simulink model "Athena_HIL_Test_2"  (R2024b)
settings: Solver=FixedStepAuto  StartTime=0.0  StopTime=inf  FixedStep=0.001  RelTol=1e-3
undefined symbols (not defined in the file or in its folder): Payload
libraries: uavmavlinklib x4, dspnetwork x2, shared6dof x1
settings Model: Creator=ercu  LastModifiedBy=ercu

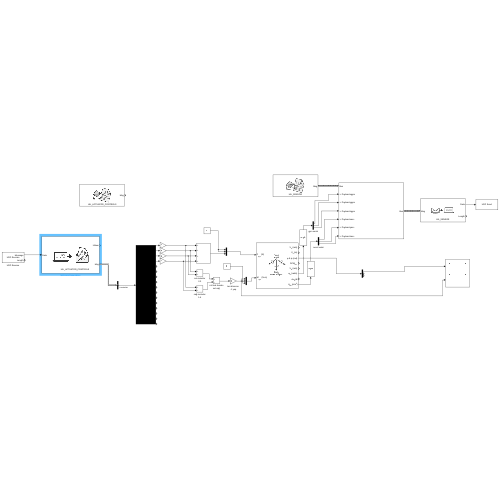
[thumbnail: Simulink's stored preview of the top-level diagram]
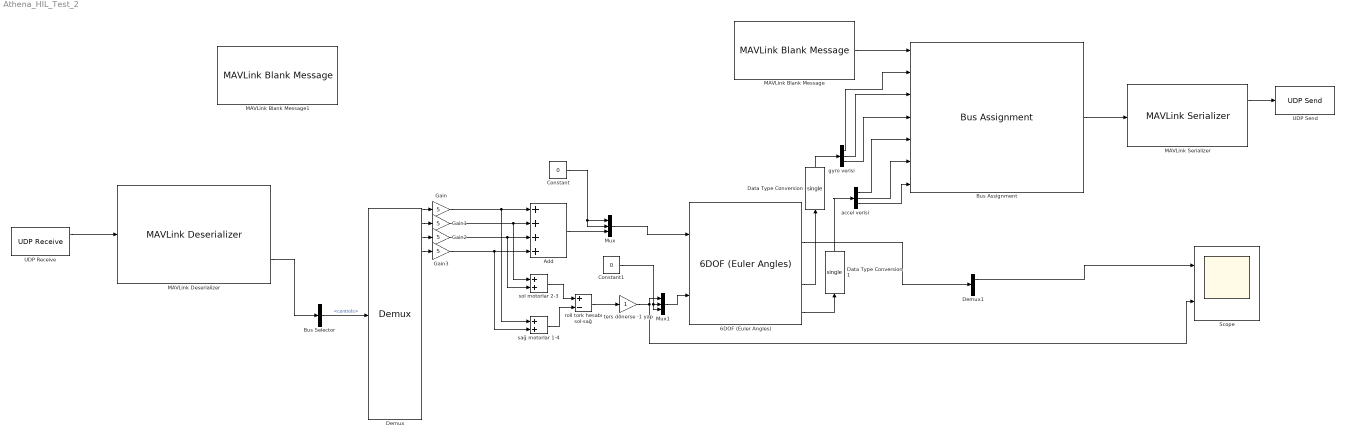
== system Athena_HIL_Test_2 ==
  6DOF (Euler Angles) : shared6dof/6DOF (Euler Angles)  units=Metric (MKS)  mtype=Fixed  rep=Euler Angles  xme_0=[0 0 -10]  Vm_0=[0 0 0]  eul_0=[0.5 0 0]  pm_0=[0 0 0]  mass_0=1.0  mass_e=0.5  mass_f=2.0  inertia=eye(3) * 0.08  inertia_e=eye(3)  inertia_f=2*eye(3)  k_quat=1.0  vre_flag=on  abi_flag=off  aMode=0  xme_statename=''  Vm_statename=''  eul_statename=''  quat_statename=''  pm_statename=''  mass_statename=''
  Add : Sum  Inputs=++++  OutDataTypeStr=double
  Bus Assignment : BusAssignment  AssignedSignals=Payload.xgyro,Payload.ygyro,Payload.zgyro,Payload.xacc,Payload.yacc,Payload.zacc
  Bus Selector : BusSelector  OutputSignals=Payload.controls
  Constant : Constant  Value=0
  Constant1 : Constant  Value=0
  Data Type Conversion : DataTypeConversion  OutDataTypeStr=single  SaturateOnIntegerOverflow=off  RndMeth=Floor
  Data Type Conversion1 : DataTypeConversion  OutDataTypeStr=single  SaturateOnIntegerOverflow=off  RndMeth=Floor
  Demux : Demux  Outputs=16
  Demux1 : Demux  Outputs=3
  Gain{,1..3} (4 alike) : Gain  Gain=5
  MAVLink Blank Message : uavmavlinklib/MAVLink Blank Message  dialectSource=Select from standard MAVLink dialects  dialect=common.xml  dialectCustom=common.xml  version=2  messageType=HIL_SENSOR  SystemID=1  ComponentID=1  SampleTime=inf
  MAVLink Blank Message1 : uavmavlinklib/MAVLink Blank Message  dialectSource=Select from standard MAVLink dialects  dialect=common.xml  dialectCustom=common.xml  version=2  messageType=HIL_ACTUATOR_CONTROLS  SystemID=1  ComponentID=1  SampleTime=inf
  MAVLink Deserializer : uavmavlinklib/MAVLink Deserializer  dialectSource=Select from standard MAVLink dialects  dialect=common.xml  dialectCustom=common.xml  version=2  messageType=HIL_ACTUATOR_CONTROLS  inputDataLength=off  SystemIDFilter=off  systemID=1  ComponentIDFilter=off  componentID=1  queueMsg=off  queueMsgSize=50  dropNum=off
  MAVLink Serializer : uavmavlinklib/MAVLink Serializer  dialectSource=Select from standard MAVLink dialects  dialect=common.xml  dialectCustom=common.xml  version=2  messageType=HIL_SENSOR
  Mux : Mux  Inputs=3
  Mux1 : Mux  Inputs=3
  Scope : Scope  NumInputPorts=2
  UDP Receive : dspnetwork/UDP Receive  localURL='0.0.0.0'  localPort=9001  remoteURL='127.0.0.1'  remotePort=-1  recvBufferSize=8192  dims=512  signalDatatype=uint8  isComplex=off  isVarSize=off  showBlockingTime=off  blockingTime=0  sampletime=0.004  blockPlatform=[]
      settings: LibrarySourceBlock=dspsrcs4/UDP Receive
  UDP Send : dspnetwork/UDP Send  remoteURL='127.0.0.1'  remotePort=9002  localURL='0.0.0.0'  localPortSource=Automatically determine  localPort=-1  sendBufferSize=8192  sampletime=-1  blockPlatform=[]  separateLengthPort=0
      settings: LibrarySourceBlock=dspsnks4/UDP Send
  accel verisi : Demux  Outputs=3
  gyro verisi : Demux  Outputs=3
  roll tork hesabı sol-sağ : Sum  Inputs=+-
  sağ motorlar 1-4 : Sum
  sol motorlar 2-3 : Sum
  ters dönerse -1 yap : Gain  OutDataTypeStr=double
  wires:
  Bus Selector/1 -> Demux/1  "<controls>"
  MAVLink Deserializer/2 -> Bus Selector/1
  UDP Receive/1 -> MAVLink Deserializer/1
  Demux/1 -> Gain/1
  Demux/2 -> Gain1/1
  Demux/3 -> Gain2/1
  Demux/4 -> Gain3/1
  Gain/1 -> sağ motorlar 1-4/1, Add/1
  Gain1/1 -> sol motorlar 2-3/1, Add/2
  Gain2/1 -> sol motorlar 2-3/2, Add/3
  Add/1 -> Mux/3
  Mux/1 -> 6DOF (Euler Angles)/1
  Constant/1 -> Mux/1, Mux/2
  Gain3/1 -> sağ motorlar 1-4/2, Add/4
  sol motorlar 2-3/1 -> roll tork hesabı sol-sağ/1
  sağ motorlar 1-4/1 -> roll tork hesabı sol-sağ/2
  roll tork hesabı sol-sağ/1 -> ters dönerse -1 yap/1
  ters dönerse -1 yap/1 -> Scope/2, Mux1/1
  Constant1/1 -> Mux1/3, Mux1/2
  Mux1/1 -> 6DOF (Euler Angles)/2
  MAVLink Blank Message/1 -> Bus Assignment/1
  MAVLink Serializer/1 -> UDP Send/1
  Bus Assignment/1 -> MAVLink Serializer/1
  6DOF (Euler Angles)/6 -> Data Type Conversion/1
  gyro verisi/1 -> Bus Assignment/2
  gyro verisi/2 -> Bus Assignment/3
  gyro verisi/3 -> Bus Assignment/4
  6DOF (Euler Angles)/8 -> Data Type Conversion1/1
  accel verisi/1 -> Bus Assignment/5
  accel verisi/2 -> Bus Assignment/6
  accel verisi/3 -> Bus Assignment/7
  6DOF (Euler Angles)/3 -> Demux1/1
  Demux1/1 -> Scope/1
  Data Type Conversion/1 -> gyro verisi/1
  Data Type Conversion1/1 -> accel verisi/1
